simulink model "simulink_interpretation"  (R2024a)
settings: Solver=VariableStepAuto  StartTime=0.0  StopTime=5  RelTol=1e-3
undefined symbols (not defined in the file): LF
libraries: instrumentseriallib x6, slrealtimeutilitieslib x2, simulink x1
settings Model: PacingRate=0.100000  Creator=osoko  LastModifiedBy=osoko

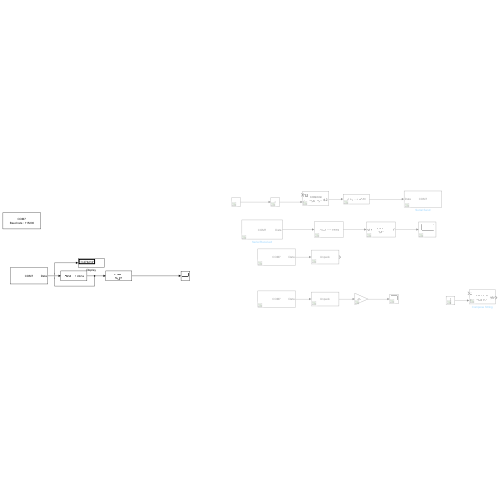
[thumbnail: Simulink's stored preview of the top-level diagram]
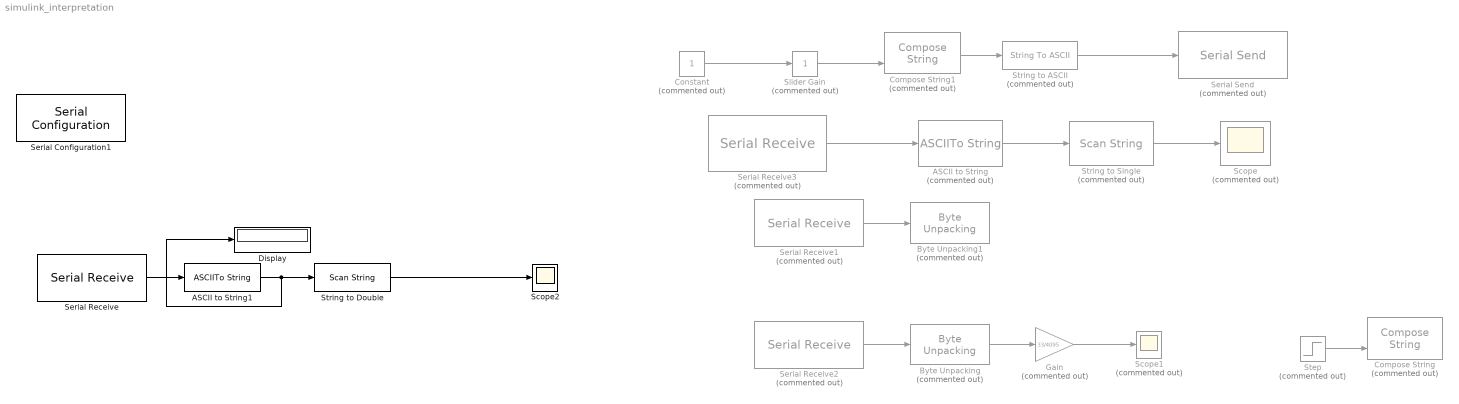
== system simulink_interpretation ==
  ASCII to String : ASCIIToString  Commented=on
  ASCII to String1 : ASCIIToString
  Byte Unpacking : slrealtimeutilitieslib/Byte Unpacking  Commented=on  MaskUnpackedDataTypes={'uint16'}  MaskUnpackedDataSizes={[1]}  MaskAlignment=2
  Byte Unpacking1 : slrealtimeutilitieslib/Byte Unpacking  Commented=on  MaskUnpackedDataTypes={'single'}  MaskUnpackedDataSizes={[1]}  MaskAlignment=4
  Compose String : ComposeString  Commented=on
  Compose String1 : ComposeString  Commented=on  Format="\"%hu %f\""
  Constant : Constant  Commented=on  OutDataTypeStr=uint32
  Display : Display
  Gain : Gain  Commented=on  Gain=33/4095  ParamDataTypeStr=single  RndMeth=Round  OutDataTypeStr=Inherit: Same as input
  Scope : Scope  Commented=on
  Scope1 : Scope  Commented=on
  Scope2 : Scope
  Serial Configuration1 : instrumentseriallib/Serial Configuration  Priority=-200000  PortSel=COM7  Port=COM7  ComPort=COM7  BaudRate=115200  DataBits=8  Parity=none  StopBits=1  ByteOrder=little-endian  FlowControl=none  Timeout=10  SimulateUsing=Interpreted execution  BlockInModel=on  aMode=1
  Serial Receive : instrumentseriallib/Serial Receive  Priority=1  PortSel=COM7  Port=COM7  ComPort=COM7  DataType=uint8  SaveDataType=uint8  ToggleHeader=off  Header=[]  ToggleDataSize=on  DataSize=[9]  ToggleTerminator=on  Terminator=LF ('\n')  CustomTerminator=[]  InputFormat=Column major  EnableBlockingMode=on  ActionDataUnavailable=Output last received value  ActionWhenDataUnavailable=Output last received value  CustomValue=0  SampleTime=0.1  SimulateUsing=Interpreted execution  BlockInModel=on  aMode=1
  Serial Receive1 : instrumentseriallib/Serial Receive  Priority=1  Commented=on  PortSel=COM7  Port=COM7  ComPort=COM7  DataType=uint8  SaveDataType=uint8  ToggleHeader=off  Header=[]  ToggleDataSize=on  DataSize=[4 1]  ToggleTerminator=on  Terminator=LF ('\n')  CustomTerminator=[]  InputFormat=Column major  EnableBlockingMode=on  ActionDataUnavailable=Output last received value  ActionWhenDataUnavailable=Output last received value  CustomValue=0  SampleTime=0.01  SimulateUsing=Interpreted execution  BlockInModel=on  aMode=1
  Serial Receive2 : instrumentseriallib/Serial Receive  Priority=1  Commented=on  PortSel=COM7  Port=COM7  ComPort=COM7  DataType=uint8  SaveDataType=uint8  ToggleHeader=off  Header=[]  ToggleDataSize=on  DataSize=[2 1]  ToggleTerminator=on  Terminator=LF ('\n')  CustomTerminator=[]  InputFormat=Column major  EnableBlockingMode=on  ActionDataUnavailable=Output last received value  ActionWhenDataUnavailable=Output last received value  CustomValue=0  SampleTime=0.01  SimulateUsing=Interpreted execution  BlockInModel=on  aMode=1
  Serial Receive3 : instrumentseriallib/Serial Receive  Priority=1  Commented=on  PortSel=COM7  Port=COM7  ComPort=COM7  DataType=uint8  SaveDataType=uint8  ToggleHeader=off  Header=[]  ToggleDataSize=on  DataSize=[9]  ToggleTerminator=on  Terminator=LF ('\n')  CustomTerminator=[]  InputFormat=Column major  EnableBlockingMode=on  ActionDataUnavailable=Output last received value  ActionWhenDataUnavailable=Output last received value  CustomValue=0  SampleTime=0.1  SimulateUsing=Interpreted execution  BlockInModel=on  aMode=1
  Serial Send : instrumentseriallib/Serial Send  Priority=1  Commented=on  PortSel=COM7  Port=COM7  ComPort=COM7  Header=[]  Terminator=LF ('\n')  CustomTerminator=[]  EnableBlockingMode=on  SimulateUsing=Interpreted execution  BlockInModel=on  aMode=1
  Slider Gain : simulink/Math Operations/Slider Gain  Commented=on  gain=1  low=0  high=999
  Step : Step  Commented=on  SampleTime=0
  String to ASCII : StringToASCII  Commented=on
  String to Double : ScanString  Format="\"%lf\""
  String to Single : ScanString  Commented=on  Format="\"%f\""
  wires:
  Byte Unpacking/1 -> Gain/1
  Serial Receive2/1 -> Byte Unpacking/1
  Gain/1 -> Scope1/1
  ASCII to String/1 -> String to Single/1
  String to Single/1 -> Scope/1
  Serial Receive1/1 -> Byte Unpacking1/1
  Serial Receive/1 -> ASCII to String1/1
  Constant/1 -> Slider Gain/1
  Slider Gain/1 -> Compose String1/2
  Compose String1/1 -> String to ASCII/1
  String to ASCII/1 -> Serial Send/1
  Step/1 -> Compose String/2
  Serial Receive3/1 -> ASCII to String/1
  ASCII to String1/1 -> Display/1, String to Double/1
  String to Double/1 -> Scope2/1
